simulink model "ModelGreenhouse"  (R2018a)
settings: Solver=FixedStepAuto  StartTime=0  StopTime=432000  FixedStep=5  RelTol=1e-1
undefined symbols (not defined in the file or in its folder): magnitude
libraries: simulink x6
(part 2 of 3)

== system ModelGreenhouse/Fogging ==
  Tair : Inport
  RH : Inport  Port=2
  I : Inport  Port=3
  Constant : Constant
  Constant1 : Constant  Value=0
  Enable : Constant  Value=0
  Integrator : Integrator
  MATLAB Function : MATLAB Function  TreatAsAtomicUnit=on
  PID Controller : simulink/Continuous/PID Controller  Controller=PI  TimeDomain=Continuous-time  SampleTime=-1  IntegratorMethod=Forward Euler  FilterMethod=Forward Euler  Form=Parallel  UseFilter=on  ControllerParametersSource=internal  P=0.005  I=0.001  D=0  N=100  InitialConditionSource=internal  InitialConditionForIntegrator=0  InitialConditionForFilter=0  ExternalReset=none  LimitOutput=off  UpperSaturationLimit=inf  LowerSaturationLimit=-inf  LinearizeAsGain=on  AntiWindupMode=none  Kb=1  TrackingMode=off  Kt=1  PParamMin=[]  PParamMax=[]  IParamMin=[]  IParamMax=[]  DParamMin=[]  DParamMax=[]  NParamMin=[]  NParamMax=[]  KbParamMin=[]  KbParamMax=[]  KtParamMin=[]  KtParamMax=[]  POutMin=[]  POutMax=[]  IOutMin=[]  IOutMax=[]  DOutMin=[]  DOutMax=[]  NOutMin=[]  NOutMax=[]  KbOutMin=[]  KbOutMax=[]  KtOutMin=[]  KtOutMax=[]  IntegratorOutMin=[]  IntegratorOutMax=[]  FilterOutMin=[]  FilterOutMax=[]  SumOutMin=[]  SumOutMax=[]  SumI1OutMin=[]  SumI1OutMax=[]  SumI2OutMin=[]  SumI2OutMax=[]  SumI3OutMin=[]  SumI3OutMax=[]  SumDOutMin=[]  SumDOutMax=[]  SaturationOutMin=[]  SaturationOutMax=[]  IntegratorContinuousStateAttributes=''  IntegratorStateMustResolveToSignalObject=off  IntegratorRTWStateStorageClass=Auto  FilterContinuousStateAttributes=''  FilterStateMustResolveToSignalObject=off  FilterRTWStateStorageClass=Auto  DifferentiatorICPrevScaledInput=0  DifferentiatorOutMin=[]  DifferentiatorOutMax=[]  FilterDiffOutCoefMin=[]  FilterDiffOutCoefMax=[]  SumDenOutMin=[]  SumDenOutMax=[]  SumNumOutMin=[]  SumNumOutMax=[]  ReciprocalOutMin=[]  ReciprocalOutMax=[]  DivideOutMin=[]  DivideOutMax=[]  TunerSelectOption=Transfer Function Based (PID Tuner App)
  Product : Product  Inputs=3
  Product1 : Product
  RH_set_Fog : Constant  Value=75
  RH_set_Fog_short : Constant  Value=75
  Rate Limiter : RateLimiter  RisingSlewLimit=1/10  FallingSlewLimit=-1/10
  Saturation : Saturate  UpperLimit=20  LowerLimit=0
  Sum : Sum  Inputs=|+-
  Switch : Switch  Criteria=u2 > Threshold  Threshold=25
  Switch1 : Switch  Criteria=u2 > Threshold  Threshold=600
  T_set_Fog : Constant  Value=25
  To Workspace : ToWorkspace  VariableName=Foggwater  SaveFormat=Timeseries  SampleTime=-1
  Phi_Fogging : Outport
  wires:
  Tair/1 -> Sum/1
  T_set_Fog/1 -> Sum/2
  Sum/1 -> Saturation/1
  Saturation/1 -> PID Controller/1
  RH/1 -> MATLAB Function/1(RH)
  MATLAB Function/1(U) -> Product/3
  I/1 -> Switch1/2, Switch/2
  Constant1/1 -> Switch/3
  Constant/1 -> Switch/1
  PID Controller/1 -> Product/2
  Switch/1 -> Product/1
  Enable/1 -> Product1/1
  Product1/1 -> Integrator/1, Phi_Fogging/1
  Product/1 -> Rate Limiter/1
  Rate Limiter/1 -> Product1/2
  Switch1/1 -> MATLAB Function/2(RHset)
  RH_set_Fog/1 -> Switch1/3
  RH_set_Fog_short/1 -> Switch1/1
  Integrator/1 -> To Workspace/1

== system ModelGreenhouse/Leak ==
  Vwind : Inport
  A_floor : Inport  Port=2
  Fcn : Fcn  Expr=3.5*u + 8.5
  Gain : Gain  Gain=1e-5
  Product : Product
  Phi_leakage : Outport
  wires:
  Vwind/1 -> Fcn/1
  Fcn/1 -> Product/1
  A_floor/1 -> Product/2
  Product/1 -> Gain/1
  Gain/1 -> Phi_leakage/1

== system ModelGreenhouse/Leakage ==
  Phi_leak : Inport
  T_out : Inport  Port=2
  T_air : Inport  Port=3
  rho_air : Inport  Port=4
  Cp : Constant  Value=1.006e3
  Product : Product  Inputs=4
  Sum : Sum  Inputs=|+-
  Q_leak : Outport
  wires:
  T_out/1 -> Sum/1
  T_air/1 -> Sum/2
  Phi_leak/1 -> Product/1
  rho_air/1 -> Product/3
  Sum/1 -> Product/2
  Product/1 -> Q_leak/1
  Cp/1 -> Product/4

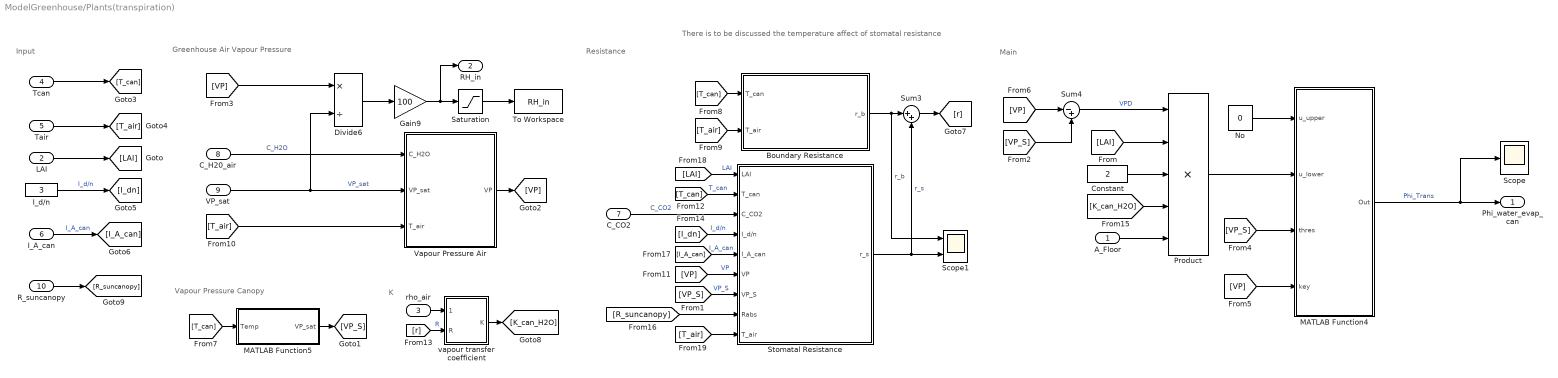
== system ModelGreenhouse/Plants(transpiration) ==
  note: There is to be discussed the temperature affect of stomatal resistance
  note: Main
  note: K
  note: Resistance
  note: Vapour Pressure Canopy
  note: Input
  note: Greenhouse Air Vapour Pressure
  A_Floor : Inport
  LAI : Inport  Port=2
  rho_air : Inport  Port=3
  Tcan : Inport  Port=4
  Tair : Inport  Port=5
  I_A_can : Inport  Port=6
  C_CO2 : Inport  Port=7
  C_H20_air : Inport  Port=8
  VP_sat : Inport  Port=9
  R_suncanopy : Inport  Port=10
  Boundary Resistance : Subsystem
  Constant : Constant  Value=2
  Divide6 : Product  Inputs=*/
  Gain9 : Gain  Gain=100
  I_d/n : Constant  Value=3
  MATLAB Function4 : MATLAB Function  TreatAsAtomicUnit=on
  MATLAB Function5 : MATLAB Function  TreatAsAtomicUnit=on
  No : Constant  Value=0
  Product : Product  Inputs=5
  Saturation : Saturate  UpperLimit=100  LowerLimit=0
  Scope : Scope
  Scope1 : Scope  NumInputPorts=2
  "Stomatal Resistance " : Subsystem
  Sum3 : Sum  Inputs=|++
  Sum4 : Sum  Inputs=|-+
  To Workspace : ToWorkspace  VariableName=RH_in  SaveFormat=Timeseries  SampleTime=-1
  Vapour Pressure Air : Subsystem
  "vapour transfer coefficient " : Subsystem
  Phi_water_evap_can : Outport
  RH_in : Outport  Port=2
  wires:
  LAI/1 -> [LAI]
  Constant/1 -> Product/3
  VP_sat/1 -> Divide6/2, Vapour Pressure Air/2(VP_sat)  "VP_sat"
  No/1 -> MATLAB Function4/1(u_upper)
  Product/1 -> MATLAB Function4/2(u_lower)
  Divide6/1 -> Gain9/1
  Gain9/1 -> Saturation/1, RH_in/1
  A_Floor/1 -> Product/5
  Sum4/1 -> Product/1  "VPD"
  [VP] -> Divide6/1
  [VP_S] -> MATLAB Function4/3(thres)
  [VP] -> MATLAB Function4/4(key)
  MATLAB Function5/1(VP_sat) -> [VP_S]
  Boundary Resistance/1(r_b) -> Scope1/1, Sum3/1  "r_b"
  Tcan/1 -> [T_can]
  [T_can] -> MATLAB Function5/1(Temp)
  [T_can] -> Boundary Resistance/1(T_can)
  Tair/1 -> [T_air]
  [T_air] -> Boundary Resistance/2(T_air)
  C_H20_air/1 -> Vapour Pressure Air/1(C_H2O)  "C_H2O"
  [T_air] -> Vapour Pressure Air/3(T_air)
  Vapour Pressure Air/1(VP) -> [VP]
  I_d/n/1 -> [I_dn]  "I_d/n"
  I_A_can/1 -> [I_A_can]  "I_A_can"
  [LAI] -> "Stomatal Resistance "/1(LAI)  "LAI"
  [T_can] -> "Stomatal Resistance "/2(T_can)  "T_can"
  C_CO2/1 -> "Stomatal Resistance "/3(C_CO2)  "C_CO2"
  [I_dn] -> "Stomatal Resistance "/4(I_d/n)  "I_d/n"
  [I_A_can] -> "Stomatal Resistance "/5(I_A_can)  "I_A_can"
  [VP] -> "Stomatal Resistance "/6(VP)  "VP"
  [VP_S] -> "Stomatal Resistance "/7(VP_S)  "VP_S"
  [LAI] -> Product/2
  Sum3/1 -> [r]
  rho_air/1 -> "vapour transfer coefficient "/1(rho_air)
  [r] -> "vapour transfer coefficient "/2(R)  "R"
  "vapour transfer coefficient "/1(K) -> [K_can_H2O]
  [K_can_H2O] -> Product/4
  [VP_S] -> Sum4/2
  [VP] -> Sum4/1
  "Stomatal Resistance "/1(r_s) -> Sum3/2, Scope1/2  "r_s"
  R_suncanopy/1 -> [R_suncanopy]
  [R_suncanopy] -> "Stomatal Resistance "/8(Rabs)
  [T_air] -> "Stomatal Resistance "/9(T_air)
  MATLAB Function4/1(Out) -> Scope/1, Phi_water_evap_can/1  "Phi_Trans"
  Saturation/1 -> To Workspace/1

== system ModelGreenhouse/Rho ==
  h_elevation : Inport
  T_air : Inport  Port=2
  Bias : Bias  Bias=273.15
  Divide : Product  Inputs=*/
  Gain : Gain  Gain=1.185
  MM_air : Constant  Value=28.96e-3
  Math Function : Math  SaturateOnIntegerOverflow=on
  Product : Product  Inputs=3
  Product1 : Product
  g : Constant  Value=9.81
  g_gas : Constant  Value=8.314
  rho_air : Outport
  wires:
  Divide/1 -> Math Function/1
  h_elevation/1 -> Product/1
  MM_air/1 -> Product/3
  Product/1 -> Divide/1
  g/1 -> Product/2
  Math Function/1 -> Gain/1
  T_air/1 -> Bias/1
  Bias/1 -> Product1/1
  g_gas/1 -> Product1/2
  Product1/1 -> Divide/2
  Gain/1 -> rho_air/1

== system ModelGreenhouse/RhoAS ==
  h_elevation : Inport
  T_airAS : Inport  Port=2
  Bias : Bias  Bias=273.15
  Divide : Product  Inputs=*/
  Gain : Gain  Gain=1.185
  MM_air : Constant  Value=28.96e-3
  Math Function : Math  SaturateOnIntegerOverflow=on
  Product : Product  Inputs=3
  Product1 : Product
  g : Constant  Value=9.81
  g_gas : Constant  Value=8.314
  rho_airAS : Outport
  wires:
  Divide/1 -> Math Function/1
  h_elevation/1 -> Product/1
  MM_air/1 -> Product/3
  Product/1 -> Divide/1
  g/1 -> Product/2
  Math Function/1 -> Gain/1
  T_airAS/1 -> Bias/1
  Bias/1 -> Product1/1
  g_gas/1 -> Product1/2
  Product1/1 -> Divide/2
  Gain/1 -> rho_airAS/1

== system ModelGreenhouse/RoofStrategy ==
  Tset_vent : Inport
  RHset_vent : Inport  Port=2
  T_air : Inport  Port=3
  RH : Inport  Port=4
  RH_out : Inport  Port=5
  I : Inport  Port=6
  Constant : Constant  Value=0
  Gain : Gain  Gain=0.6
  Gain1 : Gain  Gain=0.4
  MATLAB Function : MATLAB Function  TreatAsAtomicUnit=on
  MATLAB Function1 : MATLAB Function  TreatAsAtomicUnit=on
  Saturation : Saturate  UpperLimit=1  LowerLimit=0
  Scope : Scope
  Sum : Sum  Inputs=|++
  day/night : Switch  Threshold=20
  Uroof : Outport
  wires:
  T_air/1 -> MATLAB Function/1(T_air)
  Tset_vent/1 -> MATLAB Function/2(Tset)
  RH/1 -> MATLAB Function1/1(RH_air)
  RH_out/1 -> MATLAB Function1/2(RH_out)
  RHset_vent/1 -> MATLAB Function1/3(RH_set)
  MATLAB Function/1(y) -> Gain/1
  MATLAB Function1/1(y) -> Gain1/1
  Gain/1 -> Sum/1
  Gain1/1 -> Sum/2
  Sum/1 -> Saturation/1
  I/1 -> day/night/2
  day/night/1 -> Scope/1, Uroof/1
  Saturation/1 -> day/night/1
  Constant/1 -> day/night/3

== system ModelGreenhouse/Scr(Scr->Covin) ==
  A_floor : Inport
  T_scr : Inport  Port=2
  T_covin : Inport  Port=3
  U_Thrscr : Inport  Port=4
  " Stefan-Boltzmann constant" : Constant  Value=5.67e-8
  " epsilon_cov" : Constant  Value=0.9
  " epsilon_scr" : Constant  Value=0.44
  Bias : Bias  Bias=273.15
  Bias1 : Bias  Bias=273.15
  Fcn : Fcn  Expr=u^4
  Fcn1 : Fcn  Expr=u^4
  Product : Product  Inputs=6
  Sum : Sum  Inputs=|+-
  R_FIR_scr->covin : Outport
  wires:
  A_floor/1 -> Product/1  "A_floor"
  T_scr/1 -> Bias/1
  T_covin/1 -> Bias1/1
  Bias/1 -> Fcn/1
  Bias1/1 -> Fcn1/1
  Fcn/1 -> Sum/1
  Fcn1/1 -> Sum/2
  Sum/1 -> Product/3
  Product/1 -> R_FIR_scr->covin/1
  " Stefan-Boltzmann constant"/1 -> Product/4
  " epsilon_cov"/1 -> Product/2
  U_Thrscr/1 -> Product/5  "F"
  " epsilon_scr"/1 -> Product/6

== system ModelGreenhouse/Scr(Scr->sky) ==
  A_floor : Inport
  T_scr : Inport  Port=2
  T_sky : Inport  Port=3
  U_Thrscr : Inport  Port=4
  " Stefan-Boltzmann constant" : Constant  Value=5.67e-8
  " epsilon_scr" : Constant  Value=0.44
  " epsilon_sky" : Constant
  Bias : Bias  Bias=273.15
  Bias1 : Bias  Bias=273.15
  Fcn : Fcn  Expr=u^4
  Fcn1 : Fcn  Expr=u^4
  Product : Product  Inputs=6
  Sum : Sum  Inputs=|+-
  tau_cov : Gain  Gain=0
  R_FIR_scr->sky : Outport
  wires:
  A_floor/1 -> Product/1  "A_floor"
  T_scr/1 -> Bias/1
  T_sky/1 -> Bias1/1
  Bias/1 -> Fcn/1
  Bias1/1 -> Fcn1/1
  Fcn/1 -> Sum/1
  Fcn1/1 -> Sum/2
  Sum/1 -> Product/3
  Product/1 -> R_FIR_scr->sky/1
  " Stefan-Boltzmann constant"/1 -> Product/4
  " epsilon_sky"/1 -> Product/2
  U_Thrscr/1 -> tau_cov/1
  tau_cov/1 -> Product/5  "F"
  " epsilon_scr"/1 -> Product/6

== system ModelGreenhouse/Scr(can->scr) ==
  A_floor : Inport
  T_can : Inport  Port=2
  T_scr : Inport  Port=3
  U_Thrscr : Inport  Port=4
  LAI : Inport  Port=5
  " Stefan-Boltzmann constant" : Constant  Value=5.67e-8
  " epsilon_can" : Constant
  " epsilon_scr" : Constant  Value=0.44
  Bias : Bias  Bias=273.15
  Bias1 : Bias  Bias=273.15
  Fcn : Fcn  Expr=u^4
  Fcn1 : Fcn  Expr=u^4
  Fcn2 : Fcn  Expr=1-exp(-0.94*u)
  Product : Product  Inputs=6
  Product1 : Product
  Sum : Sum  Inputs=|+-
  R_FIR_can->scr : Outport
  wires:
  T_can/1 -> Bias/1
  T_scr/1 -> Bias1/1
  Bias/1 -> Fcn/1
  Bias1/1 -> Fcn1/1
  Fcn/1 -> Sum/1
  Fcn1/1 -> Sum/2
  Sum/1 -> Product/3
  Product/1 -> R_FIR_can->scr/1
  " Stefan-Boltzmann constant"/1 -> Product/4
  " epsilon_scr"/1 -> Product/2
  U_Thrscr/1 -> Product/5  "F"
  " epsilon_can"/1 -> Product/6
  LAI/1 -> Fcn2/1
  Product1/1 -> Product/1
  A_floor/1 -> Product1/2  "A_floor"
  Fcn2/1 -> Product1/1

== system ModelGreenhouse/Scr(floor->scr) ==
  A_floor : Inport
  T_floor : Inport  Port=2
  T_scr : Inport  Port=3
  U_Thrscr : Inport  Port=4
  LAI : Inport  Port=5
  " Stefan-Boltzmann constant" : Constant  Value=5.67e-8
  " epsilon_floor" : Constant
  " epsilon_scr" : Constant  Value=0.44
  Bias : Bias  Bias=273.15
  Bias1 : Bias  Bias=273.15
  Fcn : Fcn  Expr=u^4
  Fcn1 : Fcn  Expr=u^4
  Fcn2 : Fcn  Expr=exp(-0.94*u)
  Product : Product  Inputs=6
  Product1 : Product
  Sum : Sum  Inputs=|+-
  R_FIR_floor->scr : Outport
  wires:
  T_floor/1 -> Bias/1
  T_scr/1 -> Bias1/1
  Bias/1 -> Fcn/1
  Bias1/1 -> Fcn1/1
  Fcn/1 -> Sum/1
  Fcn1/1 -> Sum/2
  Sum/1 -> Product/3
  Product/1 -> R_FIR_floor->scr/1
  " Stefan-Boltzmann constant"/1 -> Product/4
  " epsilon_scr"/1 -> Product/2
  " epsilon_floor"/1 -> Product/6
  A_floor/1 -> Product/1
  LAI/1 -> Fcn2/1
  Product1/1 -> Product/5
  Fcn2/1 -> Product1/1
  U_Thrscr/1 -> Product1/2

== system ModelGreenhouse/ScrB(Condensation) ==
  A_Scr : Inport
  T_air : Inport  Port=2
  T_scr : Inport  Port=3
  C_H2O_air : Inport  Port=4
  rho_air : Inport  Port=5
  VP_Sat : Inport  Port=6
  U_Thrscr : Inport  Port=7
  Bias : Bias  Bias=273.15
  Constant : Constant  Value=0
  Cp_air : Constant  Value=1.006e3
  Divide1 : Product  Inputs=*/
  Fcn : Fcn  Expr=3*abs(u)^0.33
  Fcn1 : Fcn  Expr=u^(2/3)
  LE : Constant  Value=0.89
  MATLAB Function2 : MATLAB Function  TreatAsAtomicUnit=on
  MM_H2O : Gain  Gain=18e-3
  Product1 : Product  Inputs=4
  Product2 : Product  Inputs=4
  Rate Limiter : RateLimiter  RisingSlewLimit=5  FallingSlewLimit=-200  SampleTimeMode=inherited
  Rg : Gain  Gain=8.314
  Scope : Scope  NumInputPorts=2
  Scope2 : Scope
  Sum : Sum  Inputs=|+-
  Sum1 : Sum  Inputs=|-+
  Phi_water_cond_ThrscrB : Outport
  wires:
  T_air/1 -> Sum/1, Bias/1
  T_scr/1 -> Sum/2
  Sum/1 -> Fcn/1
  Bias/1 -> Rg/1
  Rg/1 -> Divide1/2
  rho_air/1 -> Product1/1  "rho_air"
  LE/1 -> Fcn1/1
  Fcn1/1 -> Product1/2
  Cp_air/1 -> Product1/3
  Fcn/1 -> Product1/4  "K"
  VP_Sat/1 -> MM_H2O/1  "VP_Sat"
  MM_H2O/1 -> Divide1/1
  Divide1/1 -> MATLAB Function2/3(thres), Scope/1, Sum1/1  "C_H2O_Sat"
  C_H2O_air/1 -> Scope/2, Sum1/2, MATLAB Function2/4(key)  "C_H2O_air"
  Product1/1 -> Product2/1
  A_Scr/1 -> Product2/2
  Constant/1 -> MATLAB Function2/2(u_lower)
  Product2/1 -> MATLAB Function2/1(u_upper)
  Sum1/1 -> Product2/4
  U_Thrscr/1 -> Product2/3
  MATLAB Function2/1(Out) -> Rate Limiter/1
  Rate Limiter/1 -> Scope2/1, Phi_water_cond_ThrscrB/1

== system ModelGreenhouse/ScrU(Condensation) ==
  A_Scr : Inport
  T_airAS : Inport  Port=2
  T_scr : Inport  Port=3
  C_H2O_airAS : Inport  Port=4
  rho_airAS : Inport  Port=5
  VP_SatAS : Inport  Port=6
  U_Thrscr : Inport  Port=7
  Bias : Bias  Bias=273.15
  Constant : Constant  Value=0
  Cp_air : Constant  Value=1.006e3
  Divide1 : Product  Inputs=*/
  Fcn : Fcn  Expr=3*abs(u)^0.33
  Fcn1 : Fcn  Expr=u^(2/3)
  LE : Constant  Value=0.89
  MATLAB Function2 : MATLAB Function  TreatAsAtomicUnit=on
  MM_H2O : Gain  Gain=18e-3
  Product1 : Product  Inputs=4
  Product2 : Product  Inputs=4
  Rate Limiter : RateLimiter  RisingSlewLimit=5  FallingSlewLimit=-200  SampleTimeMode=inherited
  Rg : Gain  Gain=8.314
  Scope1 : Scope  NumInputPorts=2
  Scope2 : Scope
  Sum : Sum  Inputs=|+-
  Sum1 : Sum  Inputs=|-+
  Phi_water_cond_ThrscrU : Outport
  wires:
  T_airAS/1 -> Sum/1, Bias/1
  T_scr/1 -> Sum/2
  Sum/1 -> Fcn/1
  Bias/1 -> Rg/1
  Rg/1 -> Divide1/2
  rho_airAS/1 -> Product1/1  "rho_air"
  LE/1 -> Fcn1/1
  Fcn1/1 -> Product1/2
  Cp_air/1 -> Product1/3
  Fcn/1 -> Product1/4  "K"
  VP_SatAS/1 -> MM_H2O/1  "VP_Sat"
  MM_H2O/1 -> Divide1/1
  Divide1/1 -> Scope1/1, MATLAB Function2/3(thres), Sum1/1  "C_H2O_Sat"
  C_H2O_airAS/1 -> Scope1/2, Sum1/2, MATLAB Function2/4(key)  "C_H2O_air"
  Product1/1 -> Product2/1
  A_Scr/1 -> Product2/2
  Constant/1 -> MATLAB Function2/2(u_lower)
  Product2/1 -> MATLAB Function2/1(u_upper)
  Sum1/1 -> Product2/4
  U_Thrscr/1 -> Product2/3
  MATLAB Function2/1(Out) -> Rate Limiter/1
  Rate Limiter/1 -> Scope2/1, Phi_water_cond_ThrscrU/1

== system ModelGreenhouse/Screen(Air->airAS) ==
  Phi_airASair : Inport
  T_air : Inport  Port=2
  T_airAS : Inport  Port=3
  Cp_air : Constant  Value=1.006e3
  Product : Product  Inputs=3
  Sum : Sum  Inputs=|+-
  Q_air->airAS : Outport
  wires:
  T_air/1 -> Sum/1
  T_airAS/1 -> Sum/2
  Sum/1 -> Product/3
  Cp_air/1 -> Product/1
  Phi_airASair/1 -> Product/2
  Product/1 -> Q_air->airAS/1

== system ModelGreenhouse/Screen(AirAs->scr) ==
  A_floor : Inport
  T_scr : Inport  Port=2
  T_airAS : Inport  Port=3
  U_Thrscr : Inport  Port=4
  Fcn : Fcn  Expr=1.7*abs(u)^0.33
  Product : Product  Inputs=3
  Product1 : Product
  Sum : Sum  Inputs=|+-
  Q_airAS->scr : Outport
  wires:
  T_airAS/1 -> Sum/1
  T_scr/1 -> Sum/2
  Sum/1 -> Fcn/1, Product/2
  A_floor/1 -> Product/1
  Product1/1 -> Product/3  "K"
  Fcn/1 -> Product1/1
  U_Thrscr/1 -> Product1/2
  Product/1 -> Q_airAS->scr/1

== system ModelGreenhouse/Screen(scr->air) ==
  A_floor : Inport
  T_air : Inport  Port=2
  T_scr : Inport  Port=3
  U_Thrscr : Inport  Port=4
  Fcn : Fcn  Expr=1.7*abs(u)^0.33
  Product : Product  Inputs=3
  Product1 : Product
  Sum : Sum  Inputs=|+-
  Q_scrair : Outport
  wires:
  T_scr/1 -> Sum/1
  T_air/1 -> Sum/2
  Sum/1 -> Fcn/1, Product/2
  A_floor/1 -> Product/1
  Product1/1 -> Product/3  "K"
  Fcn/1 -> Product1/1
  U_Thrscr/1 -> Product1/2
  Product/1 -> Q_scrair/1

== system ModelGreenhouse/Shading ==
  I : Inport
  Gain : Gain
  Switch : Switch  Criteria=u2 > Threshold  Threshold=600
  I_in : Outport
  wires:
  I/1 -> Switch/3, Gain/1, Switch/2
  Gain/1 -> Switch/1
  Switch/1 -> I_in/1

== system ModelGreenhouse/SideVentControl ==
  Tair : Inport
  I : Inport  Port=2
  StatusAC : Inport  Port=3
  Tout : Inport  Port=4
  Constant : Constant
  Constant1 : Constant  Value=0
  Enable : Constant
  MATLAB Function : MATLAB Function  TreatAsAtomicUnit=on
  PID Controller : simulink/Continuous/PID Controller  Controller=PID  TimeDomain=Continuous-time  SampleTime=-1  IntegratorMethod=Forward Euler  FilterMethod=Forward Euler  Form=Parallel  UseFilter=on  ControllerParametersSource=internal  P=0.25  I=1  D=0  N=100  InitialConditionSource=internal  InitialConditionForIntegrator=0  InitialConditionForFilter=0  ExternalReset=none  LimitOutput=off  UpperSaturationLimit=inf  LowerSaturationLimit=-inf  LinearizeAsGain=on  AntiWindupMode=none  Kb=1  TrackingMode=off  Kt=1  PParamMin=[]  PParamMax=[]  IParamMin=[]  IParamMax=[]  DParamMin=[]  DParamMax=[]  NParamMin=[]  NParamMax=[]  KbParamMin=[]  KbParamMax=[]  KtParamMin=[]  KtParamMax=[]  POutMin=[]  POutMax=[]  IOutMin=[]  IOutMax=[]  DOutMin=[]  DOutMax=[]  NOutMin=[]  NOutMax=[]  KbOutMin=[]  KbOutMax=[]  KtOutMin=[]  KtOutMax=[]  IntegratorOutMin=[]  IntegratorOutMax=[]  FilterOutMin=[]  FilterOutMax=[]  SumOutMin=[]  SumOutMax=[]  SumI1OutMin=[]  SumI1OutMax=[]  SumI2OutMin=[]  SumI2OutMax=[]  SumI3OutMin=[]  SumI3OutMax=[]  SumDOutMin=[]  SumDOutMax=[]  SaturationOutMin=[]  SaturationOutMax=[]  IntegratorContinuousStateAttributes=''  IntegratorStateMustResolveToSignalObject=off  IntegratorRTWStateStorageClass=Auto  FilterContinuousStateAttributes=''  FilterStateMustResolveToSignalObject=off  FilterRTWStateStorageClass=Auto  DifferentiatorICPrevScaledInput=0  DifferentiatorOutMin=[]  DifferentiatorOutMax=[]  FilterDiffOutCoefMin=[]  FilterDiffOutCoefMax=[]  SumDenOutMin=[]  SumDenOutMax=[]  SumNumOutMin=[]  SumNumOutMax=[]  ReciprocalOutMin=[]  ReciprocalOutMax=[]  DivideOutMin=[]  DivideOutMax=[]  TunerSelectOption=Transfer Function Based (PID Tuner App)
  Product : Product  Inputs=3
  Saturation : Saturate  UpperLimit=30  LowerLimit=0
  Saturation1 : Saturate  UpperLimit=1  LowerLimit=0
  Sum : Sum  Inputs=|+-
  Switch : Switch  Criteria=u2 > Threshold  Threshold=20
  T_set : Constant  Value=25
  U_Sidewin : Outport
  wires:
  Tair/1 -> MATLAB Function/3(Tin), Sum/1
  T_set/1 -> Sum/2
  Sum/1 -> Saturation/1
  Saturation/1 -> PID Controller/1
  PID Controller/1 -> Saturation1/1
  Product/1 -> U_Sidewin/1
  Constant/1 -> Switch/1
  Switch/1 -> Product/3
  I/1 -> Switch/2
  Constant1/1 -> Switch/3
  StatusAC/1 -> MATLAB Function/4(Status)
  Tout/1 -> MATLAB Function/2(Tout)
  Enable/1 -> MATLAB Function/1(Enable)
  MATLAB Function/1(y) -> Product/1
  Saturation1/1 -> Product/2

== system ModelGreenhouse/Sidewindow ==
  A_sidewindow : Inport
  V_wind : Inport  Port=2
  U_sidew : Inport  Port=3
  Cd : Constant  Value=0.75
  Cw : Constant  Value=0.9
  Fcn : Fcn  Expr=u*(2-u)
  Gain : Gain  Gain=1/2
  Product : Product  Inputs=4
  Product1 : Product  Inputs=3
  Sqrt : Sqrt  SaturateOnIntegerOverflow=on
  epli : Constant  Value=0.33
  Phi_Sidewindow : Outport
  wires:
  A_sidewindow/1 -> Product/1
  V_wind/1 -> Product/2
  Cd/1 -> Product/3
  Product/1 -> Gain/1
  Sqrt/1 -> Product/4
  Cw/1 -> Sqrt/1
  Gain/1 -> Product1/1
  Product1/1 -> Phi_Sidewindow/1
  U_sidew/1 -> Product1/2
  Fcn/1 -> Product1/3
  epli/1 -> Fcn/1

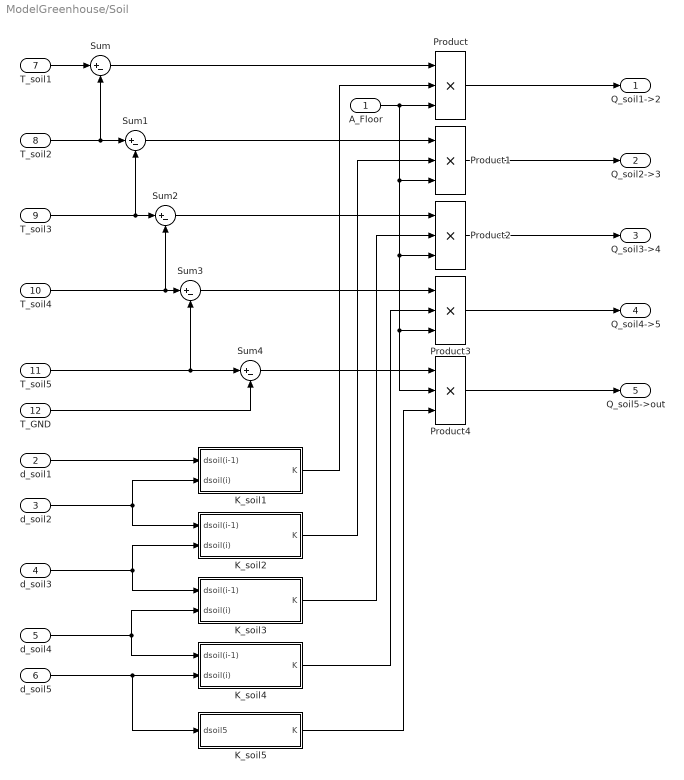
== system ModelGreenhouse/Soil ==
  A_Floor : Inport
  d_soil1 : Inport  Port=2
  d_soil2 : Inport  Port=3
  d_soil3 : Inport  Port=4
  d_soil4 : Inport  Port=5
  d_soil5 : Inport  Port=6
  T_soil1 : Inport  Port=7
  T_soil2 : Inport  Port=8
  T_soil3 : Inport  Port=9
  T_soil4 : Inport  Port=10
  T_soil5 : Inport  Port=11
  T_GND : Inport  Port=12
  K_soil1 : Subsystem
  K_soil2 : Subsystem
  K_soil3 : Subsystem
  K_soil4 : Subsystem
  K_soil5 : Subsystem
  Product{,1..4} (5 alike) : Product  Inputs=3
  Sum{,1..4} (5 alike) : Sum  Inputs=|+-
  Q_soil1->2 : Outport
  Q_soil2->3 : Outport  Port=2
  Q_soil3->4 : Outport  Port=3
  Q_soil4->5 : Outport  Port=4
  Q_soil5->out : Outport  Port=5
  wires:
  d_soil2/1 -> K_soil1/2(dsoil(i)), K_soil2/1(dsoil(i-1))
  d_soil1/1 -> K_soil1/1(dsoil(i-1))
  d_soil3/1 -> K_soil3/1(dsoil(i-1)), K_soil2/2(dsoil(i))
  d_soil4/1 -> K_soil3/2(dsoil(i)), K_soil4/1(dsoil(i-1))
  d_soil5/1 -> K_soil5/1(dsoil5), K_soil4/2(dsoil(i))
  T_soil1/1 -> Sum/1
  T_soil2/1 -> Sum/2, Sum1/1
  Sum/1 -> Product/1
  K_soil1/1(K) -> Product/2
  A_Floor/1 -> Product2/3, Product4/2, Product3/3, Product1/3, Product/3
  Product/1 -> Q_soil1->2/1
  Sum1/1 -> Product1/1
  K_soil2/1(K) -> Product1/2
  Product1/1 -> Q_soil2->3/1
  T_soil3/1 -> Sum2/1, Sum1/2
  Sum2/1 -> Product2/1
  T_soil4/1 -> Sum3/1, Sum2/2
  Sum3/1 -> Product3/1
  K_soil3/1(K) -> Product2/2
  T_soil5/1 -> Sum3/2, Sum4/1
  K_soil4/1(K) -> Product3/2
  Product2/1 -> Q_soil3->4/1
  Product3/1 -> Q_soil4->5/1
  T_GND/1 -> Sum4/2
  Sum4/1 -> Product4/1
  K_soil5/1(K) -> Product4/3
  Product4/1 -> Q_soil5->out/1

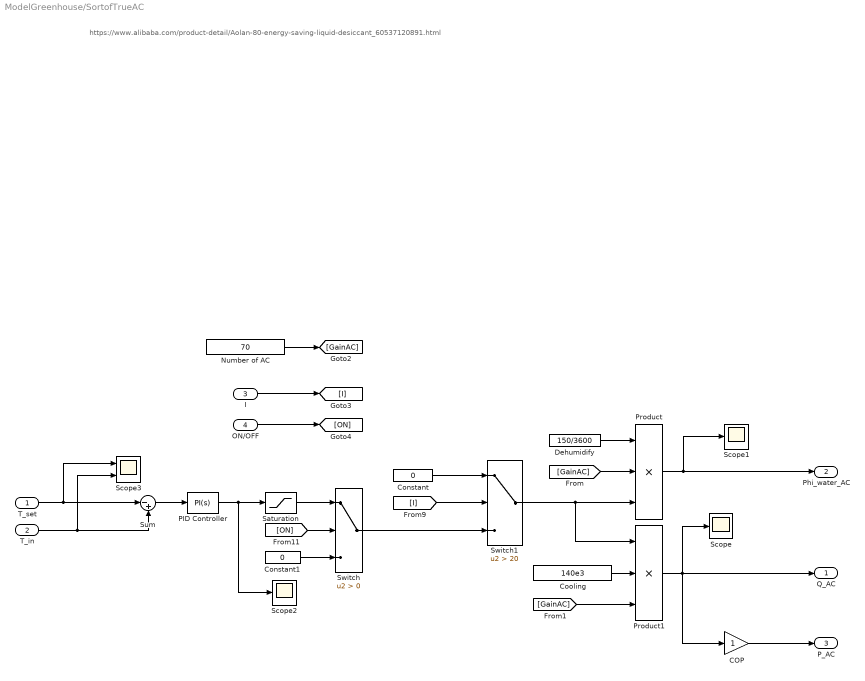
== system ModelGreenhouse/SortofTrueAC ==
  note: https://www.alibaba.com/product-detail/Aolan-80-energy-saving-liquid-desiccant_60537120891.html
  T_set : Inport
  T_in : Inport  Port=2
  I : Inport  Port=3
  ON/OFF : Inport  Port=4
  COP : Gain
  Constant : Constant  Value=0
  Constant1 : Constant  Value=0
  Cooling : Constant  Value=140e3
  Dehumidify : Constant  Value=150/3600
  Number of AC : Constant  Value=70
  PID Controller : simulink/Continuous/PID Controller  Controller=PI  TimeDomain=Continuous-time  SampleTime=-1  IntegratorMethod=Forward Euler  FilterMethod=Forward Euler  Form=Parallel  UseFilter=on  ControllerParametersSource=internal  P=1.1  I=0.000001  D=0  N=100  InitialConditionSource=internal  InitialConditionForIntegrator=0  InitialConditionForFilter=0  ExternalReset=none  LimitOutput=off  UpperSaturationLimit=inf  LowerSaturationLimit=-inf  LinearizeAsGain=on  AntiWindupMode=none  Kb=1  TrackingMode=off  Kt=1  PParamMin=[]  PParamMax=[]  IParamMin=[]  IParamMax=[]  DParamMin=[]  DParamMax=[]  NParamMin=[]  NParamMax=[]  KbParamMin=[]  KbParamMax=[]  KtParamMin=[]  KtParamMax=[]  POutMin=[]  POutMax=[]  IOutMin=[]  IOutMax=[]  DOutMin=[]  DOutMax=[]  NOutMin=[]  NOutMax=[]  KbOutMin=[]  KbOutMax=[]  KtOutMin=[]  KtOutMax=[]  IntegratorOutMin=[]  IntegratorOutMax=[]  FilterOutMin=[]  FilterOutMax=[]  SumOutMin=[]  SumOutMax=[]  SumI1OutMin=[]  SumI1OutMax=[]  SumI2OutMin=[]  SumI2OutMax=[]  SumI3OutMin=[]  SumI3OutMax=[]  SumDOutMin=[]  SumDOutMax=[]  SaturationOutMin=[]  SaturationOutMax=[]  IntegratorContinuousStateAttributes=''  IntegratorStateMustResolveToSignalObject=off  IntegratorRTWStateStorageClass=Auto  FilterContinuousStateAttributes=''  FilterStateMustResolveToSignalObject=off  FilterRTWStateStorageClass=Auto  DifferentiatorICPrevScaledInput=0  DifferentiatorOutMin=[]  DifferentiatorOutMax=[]  FilterDiffOutCoefMin=[]  FilterDiffOutCoefMax=[]  SumDenOutMin=[]  SumDenOutMax=[]  SumNumOutMin=[]  SumNumOutMax=[]  ReciprocalOutMin=[]  ReciprocalOutMax=[]  DivideOutMin=[]  DivideOutMax=[]  TunerSelectOption=Transfer Function Based (PID Tuner App)
  Product : Product  Inputs=3
  Product1 : Product  Inputs=3
  Saturation : Saturate  UpperLimit=1  LowerLimit=0
  Scope : Scope
  Scope1 : Scope
  Scope2 : Scope
  Scope3 : Scope  NumInputPorts=2
  Sum : Sum  Inputs=|-+
  Switch : Switch  Criteria=u2 > Threshold
  Switch1 : Switch  Criteria=u2 > Threshold  Threshold=20
  Q_AC : Outport
  Phi_water_AC : Outport  Port=2
  P_AC : Outport  Port=3
  wires:
  T_set/1 -> Scope3/1, Sum/1
  T_in/1 -> Scope3/2, Sum/2
  Sum/1 -> PID Controller/1
  PID Controller/1 -> Scope2/1, Saturation/1
  Constant/1 -> Switch1/1
  Switch/1 -> Switch1/3
  Saturation/1 -> Switch/1
  Constant1/1 -> Switch/3
  Number of AC/1 -> [GainAC]
  I/1 -> [I]
  [I] -> Switch1/2
  ON/OFF/1 -> [ON]
  [ON] -> Switch/2
  Dehumidify/1 -> Product/1
  Switch1/1 -> Product1/1, Product/3
  [GainAC] -> Product/2
  Product/1 -> Scope1/1, Phi_water_AC/1
  Cooling/1 -> Product1/2
  [GainAC] -> Product1/3
  Product1/1 -> COP/1, Scope/1, Q_AC/1
  COP/1 -> P_AC/1

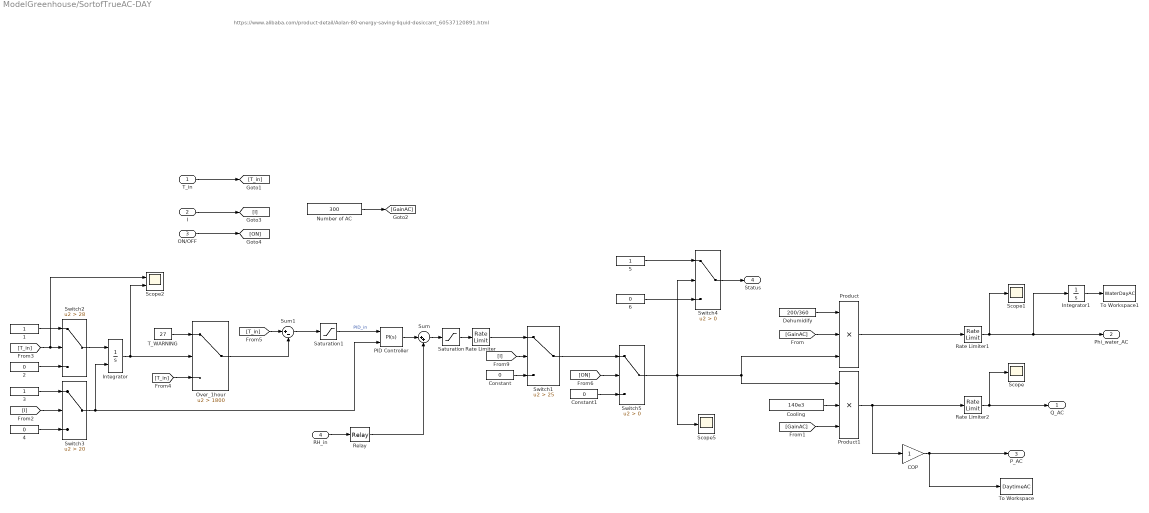
== system ModelGreenhouse/SortofTrueAC-DAY ==
  note: https://www.alibaba.com/product-detail/Aolan-80-energy-saving-liquid-desiccant_60537120891.html
  T_in : Inport
  I : Inport  Port=2
  ON/OFF : Inport  Port=3
  RH_in : Inport  Port=4
  1 : Constant
  2 : Constant  Value=0
  3 : Constant
  4 : Constant  Value=0
  5 : Constant
  6 : Constant  Value=0
  COP : Gain
  Constant : Constant  Value=0
  Constant1 : Constant  Value=0
  Cooling : Constant  Value=140e3
  Dehumidify : Constant  Value=200/360
  Integrator : Integrator  ExternalReset=rising
  Integrator1 : Integrator
  Number of AC : Constant  Value=300
  Over_1hour : Switch  Criteria=u2 > Threshold  Threshold=1800
  PID Controller : simulink/Continuous/PID Controller  Controller=PI  TimeDomain=Continuous-time  SampleTime=-1  IntegratorMethod=Forward Euler  FilterMethod=Forward Euler  Form=Parallel  UseFilter=on  ControllerParametersSource=internal  P=0.5  I=0  D=0  N=100  InitialConditionSource=internal  InitialConditionForIntegrator=0  InitialConditionForFilter=0  ExternalReset=rising  LimitOutput=off  UpperSaturationLimit=inf  LowerSaturationLimit=-inf  LinearizeAsGain=on  AntiWindupMode=none  Kb=1  TrackingMode=off  Kt=1  PParamMin=[]  PParamMax=[]  IParamMin=[]  IParamMax=[]  DParamMin=[]  DParamMax=[]  NParamMin=[]  NParamMax=[]  KbParamMin=[]  KbParamMax=[]  KtParamMin=[]  KtParamMax=[]  POutMin=[]  POutMax=[]  IOutMin=[]  IOutMax=[]  DOutMin=[]  DOutMax=[]  NOutMin=[]  NOutMax=[]  KbOutMin=[]  KbOutMax=[]  KtOutMin=[]  KtOutMax=[]  IntegratorOutMin=[]  IntegratorOutMax=[]  FilterOutMin=[]  FilterOutMax=[]  SumOutMin=[]  SumOutMax=[]  SumI1OutMin=[]  SumI1OutMax=[]  SumI2OutMin=[]  SumI2OutMax=[]  SumI3OutMin=[]  SumI3OutMax=[]  SumDOutMin=[]  SumDOutMax=[]  SaturationOutMin=[]  SaturationOutMax=[]  IntegratorContinuousStateAttributes=''  IntegratorStateMustResolveToSignalObject=off  IntegratorRTWStateStorageClass=Auto  FilterContinuousStateAttributes=''  FilterStateMustResolveToSignalObject=off  FilterRTWStateStorageClass=Auto  DifferentiatorICPrevScaledInput=0  DifferentiatorOutMin=[]  DifferentiatorOutMax=[]  FilterDiffOutCoefMin=[]  FilterDiffOutCoefMax=[]  SumDenOutMin=[]  SumDenOutMax=[]  SumNumOutMin=[]  SumNumOutMax=[]  ReciprocalOutMin=[]  ReciprocalOutMax=[]  DivideOutMin=[]  DivideOutMax=[]  TunerSelectOption=Transfer Function Based (PID Tuner App)
  Product : Product  Inputs=3
  Product1 : Product  Inputs=3
  Rate Limiter : RateLimiter  RisingSlewLimit=0.1  FallingSlewLimit=-0.1  SampleTimeMode=inherited
  Rate Limiter1 : RateLimiter  SampleTimeMode=inherited
  Rate Limiter2 : RateLimiter  RisingSlewLimit=2e7/50  FallingSlewLimit=-2e7/50  SampleTimeMode=inherited
  Relay : Relay  OnSwitchValue=96  OffSwitchValue=94
  Saturation : Saturate  UpperLimit=1  LowerLimit=0
  Saturation1 : Saturate  UpperLimit=100  LowerLimit=0
  Scope : Scope
  Scope1 : Scope
  Scope2 : Scope  NumInputPorts=2
  Scope5 : Scope
  Sum : Sum  Inputs=|++
  Sum1 : Sum  Inputs=|+-
  Switch1 : Switch  Criteria=u2 > Threshold  Threshold=25
  Switch2 : Switch  Criteria=u2 > Threshold  Threshold=28
  Switch3 : Switch  Criteria=u2 > Threshold  Threshold=20
  Switch4 : Switch  Criteria=u2 > Threshold
  Switch5 : Switch  Criteria=u2 > Threshold
  T_WARNING : Constant  Value=27
  To Workspace : ToWorkspace  VariableName=DaytimeAC  SaveFormat=Timeseries  SampleTime=-1
  To Workspace1 : ToWorkspace  VariableName=WaterDayAC  SaveFormat=Timeseries  SampleTime=-1
  Q_AC : Outport
  Phi_water_AC : Outport  Port=2
  P_AC : Outport  Port=3
  Status : Outport  Port=4
  wires:
  Number of AC/1 -> [GainAC]
  I/1 -> [I]
  ON/OFF/1 -> [ON]
  Dehumidify/1 -> Product/1
  [GainAC] -> Product/2
  Product/1 -> Rate Limiter1/1
  Cooling/1 -> Product1/2
  [GainAC] -> Product1/3
  Product1/1 -> Rate Limiter2/1, COP/1
  COP/1 -> To Workspace/1, P_AC/1
  [I] -> Switch1/2
  Constant/1 -> Switch1/3
  1/1 -> Switch2/1
  2/1 -> Switch2/3
  Switch2/1 -> Integrator/1
  3/1 -> Switch3/1
  4/1 -> Switch3/3
  [I] -> Switch3/2
  Switch3/1 -> PID Controller/2, Integrator/2
  Integrator/1 -> Over_1hour/2, Scope2/2
  T_in/1 -> [T_in]
  [T_in] -> Scope2/1, Switch2/2
  [T_in] -> Sum1/1
  Over_1hour/1 -> Sum1/2
  Saturation1/1 -> PID Controller/1  "PID_in"
  Switch4/1 -> Status/1
  5/1 -> Switch4/1
  6/1 -> Switch4/3
  Constant1/1 -> Switch5/3
  Switch1/1 -> Switch5/1
  [ON] -> Switch5/2
  Switch5/1 -> Scope5/1, Switch4/2, Product/3, Product1/1
  Sum1/1 -> Saturation1/1
  [T_in] -> Over_1hour/3
  T_WARNING/1 -> Over_1hour/1
  Rate Limiter/1 -> Switch1/1
  Saturation/1 -> Rate Limiter/1
  Rate Limiter1/1 -> Scope1/1, Integrator1/1, Phi_water_AC/1
  Rate Limiter2/1 -> Scope/1, Q_AC/1
  PID Controller/1 -> Sum/1
  Sum/1 -> Saturation/1
  RH_in/1 -> Relay/1
  Relay/1 -> Sum/2
  Integrator1/1 -> To Workspace1/1

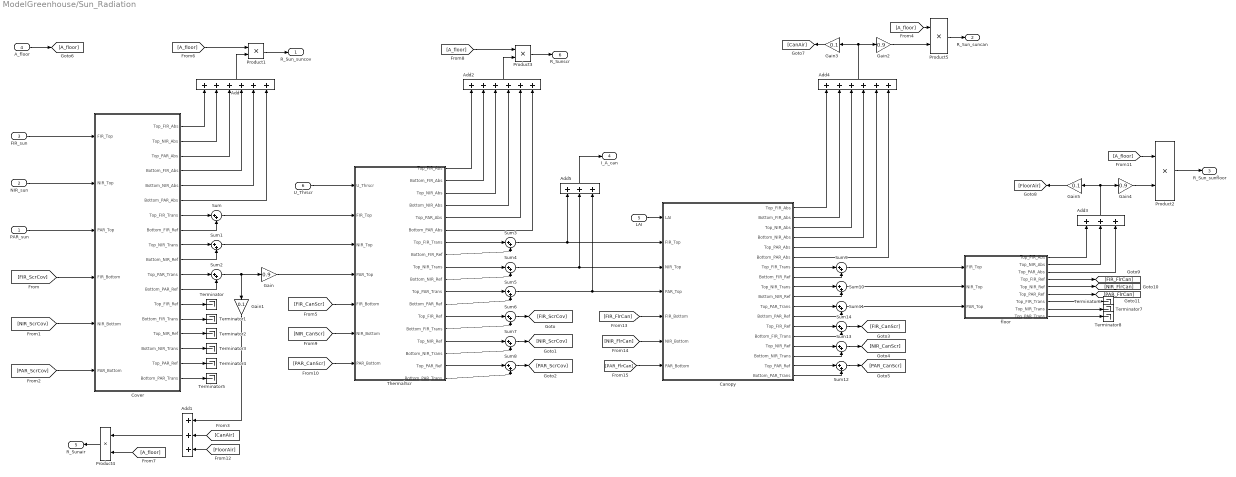
== system ModelGreenhouse/Sun_Radiation ==
  PAR_sun : Inport
  NIR_sun : Inport  Port=2
  FIR_sun : Inport  Port=3
  A_floor : Inport  Port=4
  LAI : Inport  Port=5
  U_Thrscr : Inport  Port=6
  Add : Sum  Inputs=++++++
  Add1 : Sum  Inputs=+++
  Add2 : Sum  Inputs=++++++
  Add3 : Sum  Inputs=+++
  Add4 : Sum  Inputs=++++++
  Add5 : Sum  Inputs=+++
  Canopy : Subsystem
  Cover : Subsystem
  Gain : Gain  Gain=0.9
  Gain1 : Gain  Gain=0.1
  Gain2 : Gain  Gain=0.9
  Gain3 : Gain  Gain=0.1
  Gain4 : Gain  Gain=0.9
  Gain5 : Gain  Gain=0.1
  Product{1..5} (5 alike) : Product
  Sum{,1..14} (15 alike) : Sum  Inputs=|++
  Terminator{,1..8} (9 alike) : Terminator
  ThermalScr : Subsystem
  floor : Subsystem
  R_Sun_suncov : Outport
  R_Sun_suncan : Outport  Port=2
  R_Sun_sunfloor : Outport  Port=3
  I_A_can : Outport  Port=4
  R_Sunair : Outport  Port=5
  "R_Sunscr " : Outport  Port=6
  wires:
  [FIR_ScrCov] -> Cover/4(FIR_Bottom)
  [NIR_ScrCov] -> Cover/5(NIR_Bottom)
  [PAR_ScrCov] -> Cover/6(PAR_Bottom)
  Product2/1 -> R_Sun_sunfloor/1
  [FIR_FlrCan] -> Canopy/5(FIR_Bottom)
  [NIR_FlrCan] -> Canopy/6(NIR_Bottom)
  [PAR_FlrCan] -> Canopy/7(PAR_Bottom)
  PAR_sun/1 -> Cover/3(PAR_Top)
  A_floor/1 -> [A_floor]
  LAI/1 -> Canopy/1(LAI)
  Cover/1(Top_FIR_Abs) -> Add/1
  Cover/2(Top_NIR_Abs) -> Add/2
  Cover/3(Top_PAR_Abs) -> Add/3
  Cover/4(Bottom_FIR_Abs) -> Add/4
  Cover/5(Bottom_NIR_Abs) -> Add/5
  Cover/6(Bottom_PAR_Abs) -> Add/6
  [A_floor] -> Product1/1
  Add/1 -> Product1/2
  Product1/1 -> R_Sun_suncov/1
  Cover/7(Top_FIR_Trans) -> Sum/1
  Cover/8(Bottom_FIR_Ref) -> Sum/2
  Cover/9(Top_NIR_Trans) -> Sum1/1
  Cover/10(Bottom_NIR_Ref) -> Sum1/2
  Cover/11(Top_PAR_Trans) -> Sum2/1
  Cover/12(Bottom_PAR_Ref) -> Sum2/2
  Sum/1 -> ThermalScr/2(FIR_Top)
  Sum1/1 -> ThermalScr/3(NIR_Top)
  Cover/13(Top_FIR_Ref) -> Terminator/1
  Cover/14(Bottom_FIR_Trans) -> Terminator1/1
  Cover/15(Top_NIR_Ref) -> Terminator2/1
  Cover/16(Bottom_NIR_Trans) -> Terminator3/1
  Cover/17(Top_PAR_Ref) -> Terminator4/1
  Cover/18(Bottom_PAR_Trans) -> Terminator5/1
  U_Thrscr/1 -> ThermalScr/1(U_Thrscr)
  NIR_sun/1 -> Cover/2(NIR_Top)
  FIR_sun/1 -> Cover/1(FIR_Top)
  Gain/1 -> ThermalScr/4(PAR_Top)
  Sum2/1 -> Gain1/1, Gain/1
  Gain1/1 -> Add1/1
  Add1/1 -> Product4/1
  [A_floor] -> Product4/2
  Product4/1 -> R_Sunair/1
  ThermalScr/1(Top_FIR_Abs) -> Add2/1
  ThermalScr/2(Bottom_FIR_Abs) -> Add2/2
  ThermalScr/3(Top_NIR_Abs) -> Add2/3
  ThermalScr/4(Bottom_NIR_Abs) -> Add2/4
  ThermalScr/5(Top_PAR_Abs) -> Add2/5
  ThermalScr/6(Bottom_PAR_Abs) -> Add2/6
  [A_floor] -> Product3/1
  Add2/1 -> Product3/2
  Product3/1 -> "R_Sunscr "/1
  ThermalScr/7(Top_FIR_Trans) -> Sum3/1
  ThermalScr/8(Bottom_FIR_Ref) -> Sum3/2
  ThermalScr/9(Top_NIR_Trans) -> Sum4/1
  ThermalScr/10(Bottom_NIR_Ref) -> Sum4/2
  ThermalScr/11(Top_PAR_Trans) -> Sum5/1
  ThermalScr/12(Bottom_PAR_Ref) -> Sum5/2
  Sum3/1 -> Add5/1, Canopy/2(FIR_Top)
  Sum4/1 -> Add5/2, Canopy/3(NIR_Top)
  Sum5/1 -> Add5/3, Canopy/4(PAR_Top)
  Sum6/1 -> [FIR_ScrCov]
  ThermalScr/13(Top_FIR_Ref) -> Sum6/1
  ThermalScr/14(Bottom_FIR_Trans) -> Sum6/2
  ThermalScr/15(Top_NIR_Ref) -> Sum7/1
  ThermalScr/16(Bottom_NIR_Trans) -> Sum7/2
  Sum7/1 -> [NIR_ScrCov]
  ThermalScr/17(Top_PAR_Ref) -> Sum8/1
  ThermalScr/18(Bottom_PAR_Trans) -> Sum8/2
  Sum8/1 -> [PAR_ScrCov]
  Canopy/1(Top_FIR_Abs) -> Add4/1
  Canopy/2(Bottom_FIR_Abs) -> Add4/2
  Canopy/3(Top_NIR_Abs) -> Add4/3
  Canopy/4(Bottom_NIR_Abs) -> Add4/4
  Canopy/5(Top_PAR_Abs) -> Add4/5
  Canopy/6(Bottom_PAR_Abs) -> Add4/6
  Add4/1 -> Gain2/1, Gain3/1
  Gain3/1 -> [CanAir]
  [CanAir] -> Add1/2
  Product5/1 -> R_Sun_suncan/1
  [A_floor] -> Product5/1
  Gain2/1 -> Product5/2
  Canopy/7(Top_FIR_Trans) -> Sum9/1
  Canopy/9(Top_NIR_Trans) -> Sum10/1
  Canopy/11(Top_PAR_Trans) -> Sum11/1
  Canopy/8(Bottom_FIR_Ref) -> Sum9/2
  Canopy/10(Bottom_NIR_Ref) -> Sum10/2
  Canopy/12(Bottom_PAR_Ref) -> Sum11/2
  Sum9/1 -> floor/1(FIR_Top)
  Sum10/1 -> floor/2(NIR_Top)
  Sum11/1 -> floor/3(PAR_Top)
  Canopy/13(Top_FIR_Ref) -> Sum14/1
  Canopy/14(Bottom_FIR_Trans) -> Sum14/2
  Canopy/15(Top_NIR_Ref) -> Sum13/1
  Canopy/16(Bottom_NIR_Trans) -> Sum13/2
  Canopy/17(Top_PAR_Ref) -> Sum12/1
  Canopy/18(Bottom_PAR_Trans) -> Sum12/2
  Add5/1 -> I_A_can/1
  Sum14/1 -> [FIR_CanScr]
  Sum13/1 -> [NIR_CanScr]
  Sum12/1 -> [PAR_CanScr]
  [FIR_CanScr] -> ThermalScr/5(FIR_Bottom)
  [NIR_CanScr] -> ThermalScr/6(NIR_Bottom)
  [PAR_CanScr] -> ThermalScr/7(PAR_Bottom)
  floor/1(Top_FIR_Abs) -> Add3/1
  floor/2(Top_NIR_Abs) -> Add3/2
  floor/3(Top_PAR_Abs) -> Add3/3
  Add3/1 -> Gain4/1, Gain5/1
  Gain4/1 -> Product2/2
  [A_floor] -> Product2/1
  Gain5/1 -> [FloorAir]
  [FloorAir] -> Add1/3
  floor/9(Top_PAR_Trans) -> Terminator8/1
  floor/8(Top_NIR_Trans) -> Terminator7/1
  floor/7(Top_FIR_Trans) -> Terminator6/1
  floor/4(Top_FIR_Ref) -> [FIR_FlrCan]
  floor/5(Top_NIR_Ref) -> [NIR_FlrCan]
  floor/6(Top_PAR_Ref) -> [PAR_FlrCan]

== system ModelGreenhouse/Vent ==
  rho_airAS : Inport
  Phi_roofvent : Inport  Port=2
  T_airAS : Inport  Port=3
  Tout : Inport  Port=4
  Cp_air : Constant  Value=1.006e3
  Product : Product  Inputs=4
  Scope3 : Scope  NumInputPorts=2
  Sum : Sum  Inputs=|+-
  Q_roofvent : Outport
  wires:
  T_airAS/1 -> Sum/1
  Tout/1 -> Sum/2
  Sum/1 -> Scope3/2, Product/4
  rho_airAS/1 -> Product/2
  Phi_roofvent/1 -> Product/3
  Cp_air/1 -> Product/1
  Product/1 -> Scope3/1, Q_roofvent/1

== system ModelGreenhouse/Vent-side ==
  rho_air : Inport
  Phi_sidevent : Inport  Port=2
  T_air : Inport  Port=3
  Tout : Inport  Port=4
  Cp_air : Constant  Value=1.006e3
  Product : Product  Inputs=4
  Scope3 : Scope  NumInputPorts=2
  Sum : Sum  Inputs=|+-
  Q_sidevent : Outport
  wires:
  T_air/1 -> Sum/1
  Tout/1 -> Sum/2
  Sum/1 -> Scope3/2, Product/4
  rho_air/1 -> Product/2
  Phi_sidevent/1 -> Product/3
  Cp_air/1 -> Product/1
  Product/1 -> Scope3/1, Q_sidevent/1

== system ModelGreenhouse/Wall(air->out) ==
  Tout : Inport
  Tair : Inport  Port=2
  U : Inport  Port=3
  A_wall : Inport  Port=4
  Gain : Gain
  Product : Product  Inputs=3
  Sum : Sum  Inputs=|+-
  Q_air->out : Outport
  wires:
  Tair/1 -> Sum/1
  Tout/1 -> Sum/2
  Sum/1 -> Product/3
  U/1 -> Product/2
  A_wall/1 -> Product/1
  Gain/1 -> Q_air->out/1
  Product/1 -> Gain/1

== system ModelGreenhouse/Water_flow(ThrScr) ==
  Phi_leakage : Inport
  C_H2O_Air : Inport  Port=2
  C_H2O_AirAs : Inport  Port=3
  Product : Product
  Sum : Sum  Inputs=|+-
  Phi_water_ThrScr : Outport
  wires:
  C_H2O_Air/1 -> Sum/1
  C_H2O_AirAs/1 -> Sum/2
  Phi_leakage/1 -> Product/1
  Sum/1 -> Product/2
  Product/1 -> Phi_water_ThrScr/1

== system ModelGreenhouse/Water_flow(leakage) ==
  Phi_leakage : Inport
  C_H2O_in : Inport  Port=2
  C_H2O_out : Inport  Port=3
  Product : Product
  Sum : Sum  Inputs=|+-
  Phi_water_leak : Outport
  wires:
  C_H2O_in/1 -> Sum/1
  C_H2O_out/1 -> Sum/2
  Phi_leakage/1 -> Product/1
  Sum/1 -> Product/2
  Product/1 -> Phi_water_leak/1

== system ModelGreenhouse/Water_flow(roofvent) ==
  Phi_roofvent : Inport
  C_H2O_AS : Inport  Port=2
  C_H2O_out : Inport  Port=3
  Product : Product
  Sum : Sum  Inputs=|+-
  Phi_water_roofvent : Outport
  wires:
  C_H2O_AS/1 -> Sum/1
  C_H2O_out/1 -> Sum/2
  Phi_roofvent/1 -> Product/1
  Sum/1 -> Product/2
  Product/1 -> Phi_water_roofvent/1

== system ModelGreenhouse/Water_flow(sidevent) ==
  Phi_sidevent : Inport
  C_H2O_air : Inport  Port=2
  C_H2O_out : Inport  Port=3
  Product : Product
  Sum : Sum  Inputs=|+-
  Phi_H2O_sidevent : Outport
  wires:
  C_H2O_air/1 -> Sum/1
  C_H2O_out/1 -> Sum/2
  Phi_sidevent/1 -> Product/1
  Sum/1 -> Product/2
  Product/1 -> Phi_H2O_sidevent/1

== system ModelGreenhouse/Plants(transpiration)/Boundary Resistance ==
  note: Different Paper give different suggestion, not senstive
  T_can : Inport
  T_air : Inport  Port=2
  Abs : Abs
  Divide1 : Product  Inputs=**/
  Fcn : Fcn  Expr=u^(2/3)
  Fcn1 : Fcn  Expr=u^(1/4)
  Gain : Gain  Gain=1147
  Gain1 : Gain  Gain=207
  Le : Constant  Value=0.89
  Lf : Constant  Value=0.055
  Manual Switch : ManualSwitch  CurrentSetting=0
  Math Function : Math  Operator=magnitude^2  SaturateOnIntegerOverflow=on
  Product2 : Product
  Sqrt : Sqrt  SaturateOnIntegerOverflow=on
  Sum : Sum  Inputs=|+-
  Sum1 : Sum  Inputs=|++
  Vair : Constant  Value=0.08
  rb : Constant  Value=100
  r_b : Outport
  wires:
  Math Function/1 -> Gain1/1
  Sqrt/1 -> Gain/1
  Vair/1 -> Math Function/1
  Fcn/1 -> Divide1/1
  Divide1/1 -> Manual Switch/1  "r_b"
  Abs/1 -> Product2/2
  Sum1/1 -> Fcn1/1
  Gain1/1 -> Sum1/2
  T_air/1 -> Sum/2
  Sum/1 -> Abs/1
  Product2/1 -> Sum1/1
  Lf/1 -> Sqrt/1, Product2/1
  Gain/1 -> Divide1/2
  Fcn1/1 -> Divide1/3
  Le/1 -> Fcn/1
  rb/1 -> Manual Switch/2
  T_can/1 -> Sum/1
  Manual Switch/1 -> r_b/1

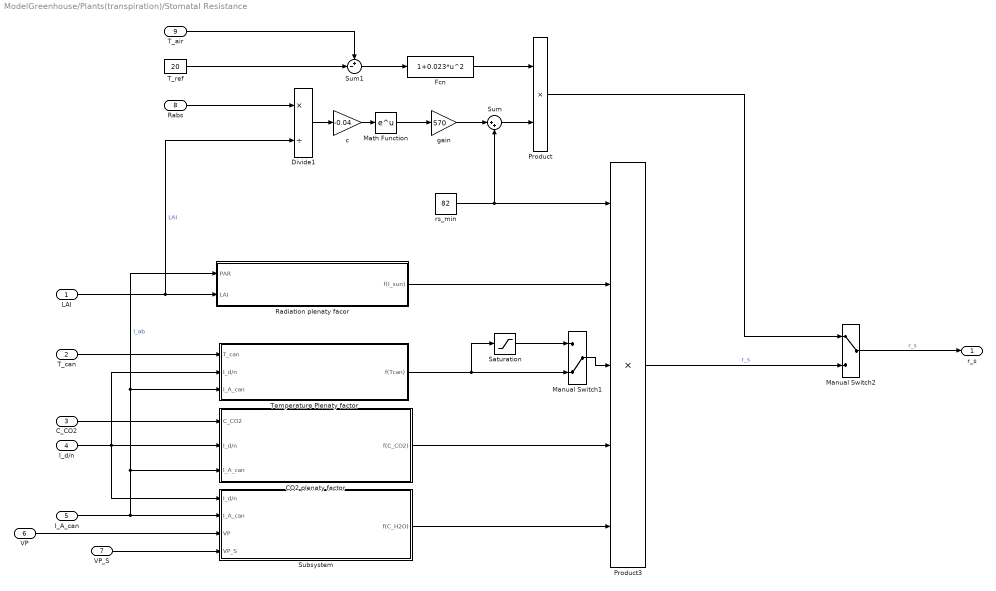
== system ModelGreenhouse/Plants(transpiration)/Stomatal Resistance  ==
  LAI : Inport
  T_can : Inport  Port=2
  C_CO2 : Inport  Port=3
  I_d/n : Inport  Port=4
  I_A_can : Inport  Port=5
  VP : Inport  Port=6
  VP_S : Inport  Port=7
  Rabs : Inport  Port=8
  T_air : Inport  Port=9
  CO2 plenaty factor : Subsystem
  Divide1 : Product  Inputs=*/
  Fcn : Fcn  Expr=1+0.023*u^2
  Manual Switch1 : ManualSwitch  CurrentSetting=0
  Manual Switch2 : ManualSwitch
  Math Function : Math  SaturateOnIntegerOverflow=on
  Product : Product
  Product3 : Product  Inputs=5
  Radiation plenaty facor : Subsystem
  Saturation : Saturate  UpperLimit=1
  Subsystem : Subsystem
  Sum : Sum  Inputs=|++
  Sum1 : Sum  Inputs=+-|
  T_ref : Constant  Value=20
  Temperature Plenaty factor : Subsystem
  c : Gain  Gain=-0.04
  gain : Gain  Gain=570
  rs_min : Constant  Value=82
  r_s : Outport
  wires:
  Manual Switch1/1 -> Product3/3
  CO2 plenaty factor/1(f(C_CO2)) -> Product3/4
  Subsystem/1(f(C_H2O)) -> Product3/5
  Radiation plenaty facor/1(f(I_sun)) -> Product3/2
  I_d/n/1 -> Subsystem/1(I_d/n), CO2 plenaty factor/2(I_d/n), Temperature Plenaty factor/2(I_d/n)
  rs_min/1 -> Sum/2, Product3/1
  Temperature Plenaty factor/1(f(Tcan)) -> Saturation/1, Manual Switch1/2
  C_CO2/1 -> CO2 plenaty factor/1(C_CO2)
  VP/1 -> Subsystem/3(VP)
  LAI/1 -> Divide1/2, Radiation plenaty facor/2(LAI)  "LAI"
  T_can/1 -> Temperature Plenaty factor/1(T_can)
  VP_S/1 -> Subsystem/4(VP_S)
  Saturation/1 -> Manual Switch1/1
  Manual Switch2/1 -> r_s/1  "r_s"
  Product3/1 -> Manual Switch2/2  "r_s"
  I_A_can/1 -> Radiation plenaty facor/1(PAR), Temperature Plenaty factor/3(I_A_can), CO2 plenaty factor/3(I_A_can), Subsystem/2(I_A_can)  "I_ab"
  Divide1/1 -> c/1
  c/1 -> Math Function/1
  Math Function/1 -> gain/1
  Rabs/1 -> Divide1/1
  gain/1 -> Sum/1
  Sum/1 -> Product/2
  Fcn/1 -> Product/1
  Product/1 -> Manual Switch2/1
  T_ref/1 -> Sum1/2
  T_air/1 -> Sum1/1
  Sum1/1 -> Fcn/1

== system ModelGreenhouse/Plants(transpiration)/Vapour Pressure Air ==
  C_H2O : Inport
  VP_sat : Inport  Port=2
  T_air : Inport  Port=3
  Divide4 : Product  Inputs=*/
  Divide5 : Product  Inputs=**/
  Fcn3 : Fcn  Expr=8.314*(u+273.15)
  Gain7 : Gain  Gain=18e-3
  VP : Outport
  wires:
  Gain7/1 -> Divide4/1
  Divide4/1 -> Divide5/3  "C_H2O_sat"
  VP_sat/1 -> Gain7/1, Divide5/2
  C_H2O/1 -> Divide5/1
  Fcn3/1 -> Divide4/2
  T_air/1 -> Fcn3/1
  Divide5/1 -> VP/1  "VP"

== system ModelGreenhouse/Plants(transpiration)/vapour transfer coefficient  ==
  rho_air : Inport
  R : Inport  Port=2
  Cp_air : Constant  Value=1.006e3
  Divide : Product  Inputs=**/
  LH : Constant  Value=2.45e6
  Product1 : Product  Inputs=3
  gamma : Constant  Value=65.8
  K : Outport
  wires:
  Cp_air/1 -> Divide/2
  gamma/1 -> Product1/2
  Product1/1 -> Divide/3
  R/1 -> Product1/3
  LH/1 -> Product1/1
  Divide/1 -> K/1  "K"
  rho_air/1 -> Divide/1

== system ModelGreenhouse/Soil/K_soil1 ==
  dsoil(i-1) : Inport
  dsoil(i) : Inport  Port=2
  Constant : Constant  Value=2
  Divide : Product  Inputs=*/
  Divide1 : Product  Inputs=*/
  Divide2 : Product  Inputs=*/
  Sum : Sum  Inputs=|++
  lambda_soil : Constant  Value=0.85
  K : Outport
  wires:
  dsoil(i-1)/1 -> Divide/1
  lambda_soil/1 -> Divide1/2, Divide/2
  dsoil(i)/1 -> Divide1/1
  Divide/1 -> Sum/1
  Divide1/1 -> Sum/2
  Sum/1 -> Divide2/2
  Constant/1 -> Divide2/1
  Divide2/1 -> K/1

== system ModelGreenhouse/Soil/K_soil2 ==
  dsoil(i-1) : Inport
  dsoil(i) : Inport  Port=2
  Constant : Constant  Value=2
  Divide : Product  Inputs=*/
  Divide1 : Product  Inputs=*/
  Divide2 : Product  Inputs=*/
  Sum : Sum  Inputs=|++
  lambda_soil : Constant  Value=0.85
  K : Outport
  wires:
  dsoil(i-1)/1 -> Divide/1
  lambda_soil/1 -> Divide1/2, Divide/2
  dsoil(i)/1 -> Divide1/1
  Divide/1 -> Sum/1
  Divide1/1 -> Sum/2
  Sum/1 -> Divide2/2
  Constant/1 -> Divide2/1
  Divide2/1 -> K/1

== system ModelGreenhouse/Soil/K_soil3 ==
  dsoil(i-1) : Inport
  dsoil(i) : Inport  Port=2
  Constant : Constant  Value=2
  Divide : Product  Inputs=*/
  Divide1 : Product  Inputs=*/
  Divide2 : Product  Inputs=*/
  Sum : Sum  Inputs=|++
  lambda_soil : Constant  Value=0.85
  K : Outport
  wires:
  dsoil(i-1)/1 -> Divide/1
  lambda_soil/1 -> Divide1/2, Divide/2
  dsoil(i)/1 -> Divide1/1
  Divide/1 -> Sum/1
  Divide1/1 -> Sum/2
  Sum/1 -> Divide2/2
  Constant/1 -> Divide2/1
  Divide2/1 -> K/1

== system ModelGreenhouse/Soil/K_soil4 ==
  dsoil(i-1) : Inport
  dsoil(i) : Inport  Port=2
  Constant : Constant  Value=2
  Divide : Product  Inputs=*/
  Divide1 : Product  Inputs=*/
  Divide2 : Product  Inputs=*/
  Sum : Sum  Inputs=|++
  lambda_soil : Constant  Value=0.85
  K : Outport
  wires:
  dsoil(i-1)/1 -> Divide/1
  lambda_soil/1 -> Divide1/2, Divide/2
  dsoil(i)/1 -> Divide1/1
  Divide/1 -> Sum/1
  Divide1/1 -> Sum/2
  Sum/1 -> Divide2/2
  Constant/1 -> Divide2/1
  Divide2/1 -> K/1

== system ModelGreenhouse/Soil/K_soil5 ==
  dsoil5 : Inport
  Constant : Constant
  Divide : Product  Inputs=*/
  Divide2 : Product  Inputs=*/
  lambda_soil : Constant  Value=0.85
  K : Outport
  wires:
  dsoil5/1 -> Divide/1
  lambda_soil/1 -> Divide/2
  Divide/1 -> Divide2/2
  Constant/1 -> Divide2/1
  Divide2/1 -> K/1

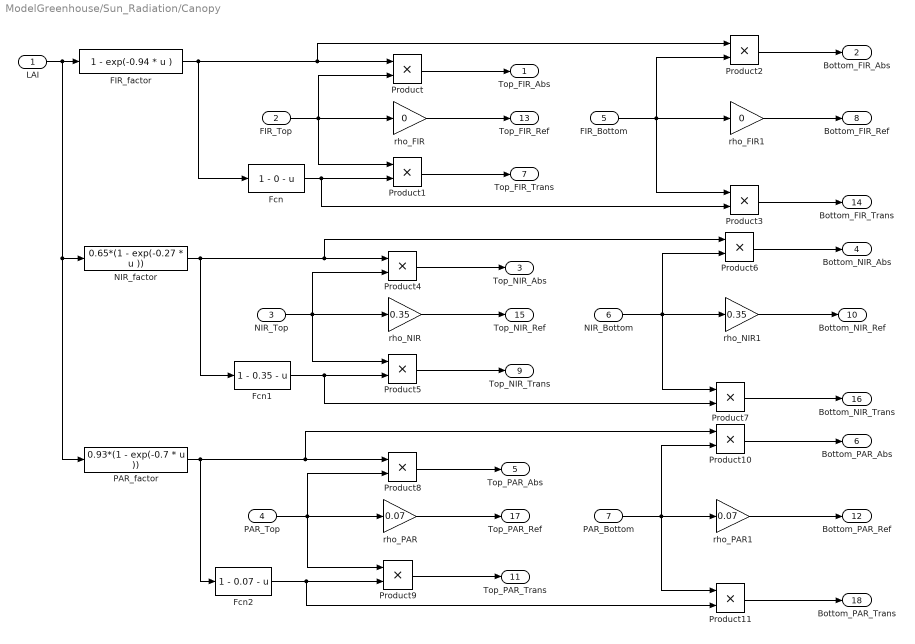
== system ModelGreenhouse/Sun_Radiation/Canopy ==
  LAI : Inport
  FIR_Top : Inport  Port=2
  NIR_Top : Inport  Port=3
  PAR_Top : Inport  Port=4
  FIR_Bottom : Inport  Port=5
  NIR_Bottom : Inport  Port=6
  PAR_Bottom : Inport  Port=7
  FIR_factor : Fcn  Expr=1 - exp(-0.94 * u )
  Fcn : Fcn  Expr=1 - 0 - u
  Fcn1 : Fcn  Expr=1 - 0.35 - u
  Fcn2 : Fcn  Expr=1 - 0.07 - u
  NIR_factor : Fcn  Expr=0.65*(1 - exp(-0.27 * u ))
  PAR_factor : Fcn  Expr=0.93*(1 - exp(-0.7 * u ))
  Product{,1..11} (12 alike) : Product
  rho_FIR : Gain  Gain=0
  rho_FIR1 : Gain  Gain=0
  rho_NIR : Gain  Gain=0.35
  rho_NIR1 : Gain  Gain=0.35
  rho_PAR : Gain  Gain=0.07
  rho_PAR1 : Gain  Gain=0.07
  Top_FIR_Abs : Outport
  Bottom_FIR_Abs : Outport  Port=2
  Top_NIR_Abs : Outport  Port=3
  Bottom_NIR_Abs : Outport  Port=4
  Top_PAR_Abs : Outport  Port=5
  Bottom_PAR_Abs : Outport  Port=6
  Top_FIR_Trans : Outport  Port=7
  Bottom_FIR_Ref : Outport  Port=8
  Top_NIR_Trans : Outport  Port=9
  Bottom_NIR_Ref : Outport  Port=10
  Top_PAR_Trans : Outport  Port=11
  Bottom_PAR_Ref : Outport  Port=12
  Top_FIR_Ref : Outport  Port=13
  Bottom_FIR_Trans : Outport  Port=14
  Top_NIR_Ref : Outport  Port=15
  Bottom_NIR_Trans : Outport  Port=16
  Top_PAR_Ref : Outport  Port=17
  Bottom_PAR_Trans : Outport  Port=18
  wires:
  Product1/1 -> Top_FIR_Trans/1
  rho_FIR/1 -> Top_FIR_Ref/1
  FIR_Top/1 -> Product1/1, Product/2, rho_FIR/1
  Product/1 -> Top_FIR_Abs/1
  FIR_Bottom/1 -> Product3/1, Product2/2, rho_FIR1/1
  rho_FIR1/1 -> Bottom_FIR_Ref/1
  Product2/1 -> Bottom_FIR_Abs/1
  rho_NIR/1 -> Top_NIR_Ref/1
  Product5/1 -> Top_NIR_Trans/1
  NIR_Top/1 -> rho_NIR/1, Product4/2, Product5/1
  Product4/1 -> Top_NIR_Abs/1
  rho_NIR1/1 -> Bottom_NIR_Ref/1
  NIR_Bottom/1 -> Product7/1, Product6/2, rho_NIR1/1
  Product6/1 -> Bottom_NIR_Abs/1
  Product7/1 -> Bottom_NIR_Trans/1
  PAR_Top/1 -> Product9/1, Product8/2, rho_PAR/1
  rho_PAR/1 -> Top_PAR_Ref/1
  Product8/1 -> Top_PAR_Abs/1
  Product11/1 -> Bottom_PAR_Trans/1
  rho_PAR1/1 -> Bottom_PAR_Ref/1
  Product10/1 -> Bottom_PAR_Abs/1
  PAR_Bottom/1 -> Product11/1, Product10/2, rho_PAR1/1
  LAI/1 -> PAR_factor/1, NIR_factor/1, FIR_factor/1
  FIR_factor/1 -> Fcn/1, Product2/1, Product/1
  Fcn/1 -> Product3/2, Product1/2
  Product3/1 -> Bottom_FIR_Trans/1
  NIR_factor/1 -> Fcn1/1, Product4/1, Product6/1
  Fcn1/1 -> Product5/2, Product7/2
  PAR_factor/1 -> Fcn2/1, Product10/1, Product8/1
  Product9/1 -> Top_PAR_Trans/1
  Fcn2/1 -> Product11/2, Product9/2

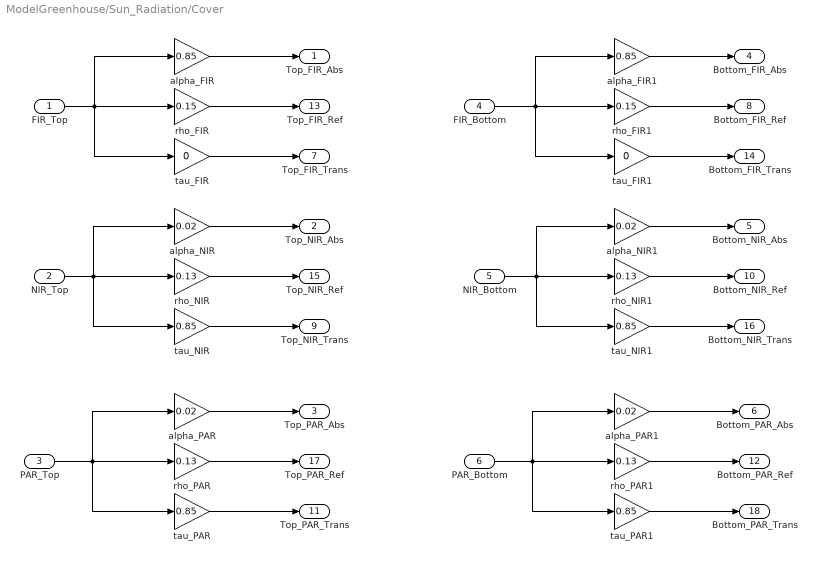
== system ModelGreenhouse/Sun_Radiation/Cover ==
  FIR_Top : Inport
  NIR_Top : Inport  Port=2
  PAR_Top : Inport  Port=3
  FIR_Bottom : Inport  Port=4
  NIR_Bottom : Inport  Port=5
  PAR_Bottom : Inport  Port=6
  alpha_FIR : Gain  Gain=0.85
  alpha_FIR1 : Gain  Gain=0.85
  alpha_NIR : Gain  Gain=0.02
  alpha_NIR1 : Gain  Gain=0.02
  alpha_PAR : Gain  Gain=0.02
  alpha_PAR1 : Gain  Gain=0.02
  rho_FIR : Gain  Gain=0.15
  rho_FIR1 : Gain  Gain=0.15
  rho_NIR : Gain  Gain=0.13
  rho_NIR1 : Gain  Gain=0.13
  rho_PAR : Gain  Gain=0.13
  rho_PAR1 : Gain  Gain=0.13
  tau_FIR : Gain  Gain=0
  tau_FIR1 : Gain  Gain=0
  tau_NIR : Gain  Gain=0.85
  tau_NIR1 : Gain  Gain=0.85
  tau_PAR : Gain  Gain=0.85
  tau_PAR1 : Gain  Gain=0.85
  Top_FIR_Abs : Outport
  Top_NIR_Abs : Outport  Port=2
  Top_PAR_Abs : Outport  Port=3
  Bottom_FIR_Abs : Outport  Port=4
  Bottom_NIR_Abs : Outport  Port=5
  Bottom_PAR_Abs : Outport  Port=6
  Top_FIR_Trans : Outport  Port=7
  Bottom_FIR_Ref : Outport  Port=8
  Top_NIR_Trans : Outport  Port=9
  Bottom_NIR_Ref : Outport  Port=10
  Top_PAR_Trans : Outport  Port=11
  Bottom_PAR_Ref : Outport  Port=12
  Top_FIR_Ref : Outport  Port=13
  Bottom_FIR_Trans : Outport  Port=14
  Top_NIR_Ref : Outport  Port=15
  Bottom_NIR_Trans : Outport  Port=16
  Top_PAR_Ref : Outport  Port=17
  Bottom_PAR_Trans : Outport  Port=18
  wires:
  tau_FIR/1 -> Top_FIR_Trans/1
  rho_FIR/1 -> Top_FIR_Ref/1
  FIR_Top/1 -> tau_FIR/1, alpha_FIR/1, rho_FIR/1
  alpha_FIR/1 -> Top_FIR_Abs/1
  FIR_Bottom/1 -> tau_FIR1/1, alpha_FIR1/1, rho_FIR1/1
  rho_FIR1/1 -> Bottom_FIR_Ref/1
  tau_FIR1/1 -> Bottom_FIR_Trans/1
  alpha_FIR1/1 -> Bottom_FIR_Abs/1
  rho_NIR/1 -> Top_NIR_Ref/1
  tau_NIR/1 -> Top_NIR_Trans/1
  NIR_Top/1 -> tau_NIR/1, rho_NIR/1, alpha_NIR/1
  alpha_NIR/1 -> Top_NIR_Abs/1
  rho_NIR1/1 -> Bottom_NIR_Ref/1
  NIR_Bottom/1 -> alpha_NIR1/1, rho_NIR1/1, tau_NIR1/1
  alpha_NIR1/1 -> Bottom_NIR_Abs/1
  tau_NIR1/1 -> Bottom_NIR_Trans/1
  tau_PAR/1 -> Top_PAR_Trans/1
  rho_PAR/1 -> Top_PAR_Ref/1
  alpha_PAR/1 -> Top_PAR_Abs/1
  PAR_Top/1 -> tau_PAR/1, alpha_PAR/1, rho_PAR/1
  tau_PAR1/1 -> Bottom_PAR_Trans/1
  rho_PAR1/1 -> Bottom_PAR_Ref/1
  alpha_PAR1/1 -> Bottom_PAR_Abs/1
  PAR_Bottom/1 -> tau_PAR1/1, alpha_PAR1/1, rho_PAR1/1
